simulink model "Sim4_LCL_L_comp_pwm"  (R2019b)
settings: Solver=ode1  StartTime=0.0  StopTime=3  FixedStep=Time_Step  MaxStep=1e-4  RelTol=1e-3
undefined symbols (not defined in the file): GRD00_Lg, GRD00_Rg, Time_Step
libraries: powerlib x13, GFo_Lib x2, Source_Lib x1, powerlib_meascontrol x1
settings Model: Creator=Frederic_Colas  LastModifiedBy=fcolas
settings DataIOCC: ReturnWorkspaceOutputs=off
settings OptimizationCC: LifeSpan=inf
settings DebuggingCC: UnconnectedInputMsg=none  UnconnectedOutputMsg=none  UnconnectedLineMsg=none  SFExecutionAtInitializationDiag=none  ArithmeticOperatorsInVariantConditions=warning
settings HardwareCC: ProdBitPerSizeT=32  ProdBitPerPtrDiffT=32  ProdWordSize=32  ProdHWDeviceType=Specified
settings SFSimCC: SimUseLocalCustomCode=off  CustomCodeUndefinedFunction=UseInterfaceOnly
settings RTWCC: RTWUseLocalCustomCode=off
settings CodeAppCC: StateflowObjectComments=on
settings SimscapeCC: SimscapeNormalizeSystem=off

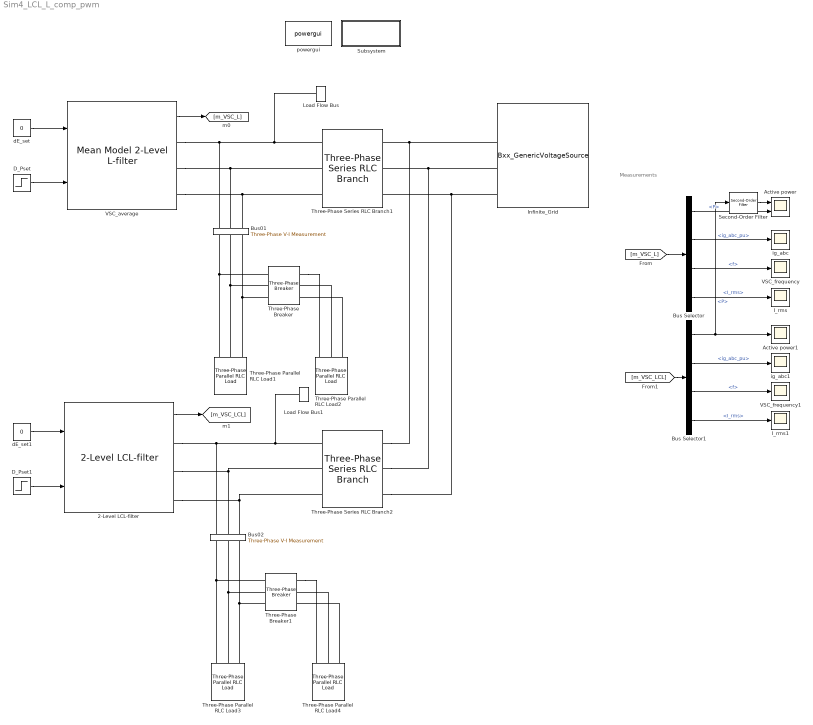
== system Sim4_LCL_L_comp_pwm ==
  note: Measurements
  2-Level LCL-filter : GFo_Lib/2-Level LCL-filter  fn=50  Sn=1000e6  Pn=1000e6  Udcn=640e3  Time_Step=Time_Step  bridge_type=Detailed (switches included)  fpwm=4.33e3  Un1=320e3  Un2=400e3  Rt_pu=0.005  Lt_pu=0.15  Rm_pu=500  Lm_pu=500  Lf_pu=0.15  Rf_pu=0.005  Cf_pu=0.066  H_DC=40  Tr_PLL=10  Val_Freq_Support=on  Val_gamma=on  R_percent=4  Rv=0.09  W_TVR=60  I_thresh_pu=1.2  DX_DR=5  Val_Mod_H=off  RLCL_D=0.7  f_damping=100  I_max_pu=1.2  Tr_I_max=200  Advanced=on  gainpopup=With Inertia  f_Inertia_Less=3  zeta_Inertia_Less=1  Param_Inertia=PI  H_GFo=5  zeta_GFo=1  LFpopup=PQ  P0=0.3  Q0=0  V0=1.0009  Theta0=0.57142
      settings: SourceProductName=VSC4SPS
  Active power : Scope  NumInputPorts=2
  Active power1 : Scope
  Bus Selector : BusSelector  OutputSignals=P,I.ig_abc_pu,f,VI.I_rms
  Bus Selector1 : BusSelector  OutputSignals=P,I.ig_abc_pu,f,VI.I_rms
  "Bus01 " : powerlib/Measurements/Three-Phase V-I Measurement  VoltageMeasurement=no  SetLabelV=off  LabelV=Vabc  Vpu=off  VpuLL=off  CurrentMeasurement=no  SetLabelI=off  LabelI=Iabc  Ipu=off  Pbase=100e6  Vbase=500e3  OutputType=Complex  PhasorSimulation=off  PSBequivalent=0
  Bus02 : powerlib/Measurements/Three-Phase V-I Measurement  VoltageMeasurement=no  SetLabelV=off  LabelV=Vabc  Vpu=off  VpuLL=off  CurrentMeasurement=no  SetLabelI=off  LabelI=Iabc  Ipu=off  Pbase=100e6  Vbase=500e3  OutputType=Complex  PhasorSimulation=off  PSBequivalent=0
  D_Pset : Step  Time=0.25  After=0.6  SampleTime=0
  D_Pset1 : Step  Time=0.25  After=0.6  SampleTime=0
  I_rms : Scope
  I_rms1 : Scope
  Infinite_Grid : Source_Lib/Bxx_GenericVoltageSource  SourceNature_str=INFINITE  fn=50  Sn=1000e6  Un=Ug  Time_Step=0  LFpopup=Swing  P0=-398902388.0153  Q0=3978449.8636  V0_pu=1  U0=20000  Theta0_deg=0  H_s=5  DroopOnOff=on  R_percent=4  TN=1  TD=2
      settings: SourceProductName=VSC4SPS
  Load Flow Bus : powerlib/Measurements/Load Flow Bus  LConnTagsString=a  Phases=single  Connectors=on one side  ID=BUS_1  Vbase=Ug  Vref=1  Vangle=0  VLF=1.001  VLFb=1  VLFc=1  angleLF=0.5714  angleLFb=0  angleLFc=0
  Load Flow Bus1 : powerlib/Measurements/Load Flow Bus  LConnTagsString=a  Phases=single  Connectors=on one side  ID=BUS_2  Vbase=Ug  Vref=1  Vangle=0  VLF=1.001  VLFb=1  VLFc=1  angleLF=0.5714  angleLFb=0  angleLFc=0
  Second-Order Filter : powerlib_meascontrol/Filters/Second-Order Filter  FilterType=Lowpass  Fo=250  Zeta=1  Ts=0  Initialize=on  Vac_Init="[0,  0,  60]"  Vdc_Init=0.3  PlotResponse=off  FreqRange=[0, 500, 1]
      settings: SourceProductBaseCode=PS
  Subsystem : Subsystem
      settings: OpenFcn=LoadFlow_VSC
      mask Display: color('blue'),disp('Update Loadflow')
  Three-Phase Parallel RLC Load1 : powerlib/Elements/Three-Phase Parallel RLC Load  LConnTagsString=A|B|C  Configuration=Y (grounded)  NominalVoltage=Ug  Vabc=[1e3 1e3 1e3]  Vabcp=[1e3 1e3 1e3]  NominalFrequency=fb  UnbalancedPower=off  ActivePower=100e6  InductivePower=0  CapacitivePower=0  Pabc=[10e3 9e3 11e3]  QLabc=[100 90 110]  QCabc=[100 90 110]  Pabcp=[10e3 9e3 11e3]  QLabcp=[100 90 110]  QCabcp=[100 90 110]  Measurements=None  LoadType=constant Z
  Three-Phase Parallel RLC Load2 : powerlib/Elements/Three-Phase Parallel RLC Load  LConnTagsString=A|B|C  Configuration=Y (grounded)  NominalVoltage=Ug  Vabc=[1e3 1e3 1e3]  Vabcp=[1e3 1e3 1e3]  NominalFrequency=fb  UnbalancedPower=off  ActivePower=1000e6  InductivePower=0  CapacitivePower=0  Pabc=[10e3 9e3 11e3]  QLabc=[100 90 110]  QCabc=[100 90 110]  Pabcp=[10e3 9e3 11e3]  QLabcp=[100 90 110]  QCabcp=[100 90 110]  Measurements=None  LoadType=constant Z
  Three-Phase Parallel RLC Load3 : powerlib/Elements/Three-Phase Parallel RLC Load  LConnTagsString=A|B|C  Configuration=Y (grounded)  NominalVoltage=Ug  Vabc=[1e3 1e3 1e3]  Vabcp=[1e3 1e3 1e3]  NominalFrequency=fb  UnbalancedPower=off  ActivePower=100e6  InductivePower=0  CapacitivePower=0  Pabc=[10e3 9e3 11e3]  QLabc=[100 90 110]  QCabc=[100 90 110]  Pabcp=[10e3 9e3 11e3]  QLabcp=[100 90 110]  QCabcp=[100 90 110]  Measurements=None  LoadType=constant Z
  Three-Phase Parallel RLC Load4 : powerlib/Elements/Three-Phase Parallel RLC Load  LConnTagsString=A|B|C  Configuration=Y (grounded)  NominalVoltage=Ug  Vabc=[1e3 1e3 1e3]  Vabcp=[1e3 1e3 1e3]  NominalFrequency=fb  UnbalancedPower=off  ActivePower=1000e6  InductivePower=0  CapacitivePower=0  Pabc=[10e3 9e3 11e3]  QLabc=[100 90 110]  QCabc=[100 90 110]  Pabcp=[10e3 9e3 11e3]  QLabcp=[100 90 110]  QCabcp=[100 90 110]  Measurements=None  LoadType=constant Z
  Three-Phase Series RLC Branch1 : powerlib/Elements/Three-Phase Series RLC Branch  LConnTagsString=A|B|C  RConnTagsString=A|B|C  BranchType=RL  Resistance=GRD00_Rg  Inductance=GRD00_Lg  Capacitance=1e-6  Measurements=None
  Three-Phase Series RLC Branch2 : powerlib/Elements/Three-Phase Series RLC Branch  LConnTagsString=A|B|C  RConnTagsString=A|B|C  BranchType=RL  Resistance=GRD00_Rg  Inductance=GRD00_Lg  Capacitance=1e-6  Measurements=None
  Three-Phase Breaker : powerlib/Elements/Three-Phase Breaker  InitialState=open  SwitchA=on  SwitchB=on  SwitchC=on  SwitchTimes=1  External=off  BreakerResistance=0.01  SnubberResistance=1e6  SnubberCapacitance=inf  Measurements=None
  Three-Phase Breaker1 : powerlib/Elements/Three-Phase Breaker  InitialState=open  SwitchA=on  SwitchB=on  SwitchC=on  SwitchTimes=1  External=off  BreakerResistance=0.01  SnubberResistance=1e6  SnubberCapacitance=inf  Measurements=None
  VSC_average : GFo_Lib/Mean Model 2-Level L-filter  fn=50  Sn=1000e6  Pn=1000e6  Udcn=640e3  Time_Step=Time_Step  Un1=320e3  Un2=Ug  Rt_pu=0.005  Lt_pu=0.15  Lm_pu=500  Rm_pu=500  Tr_PLL=10  Val_Freq_Support=on  R_percent=4  Rv=0.09  W_TVR=60  I_max_VI_pu=1.2  DX_DR=5  Val_Mod_H=off  I_max_pu=1.2  Tr_I_max=200  Advanced=on  gainpopup=With Inertia  f_Inertia_Less=5  zeta_Inertia_Less=1  Param_Inertia=PI  H_GFo=5  zeta_GFo=1  LFpopup=PQ  P0=0.3  Q0=2.3716e-08  V0=1.0009  Theta0=0.57142
      settings: SourceProductName=VSC4SPS
  VSC_frequency : Scope
  VSC_frequency1 : Scope
  dE_set : Constant  Value=0
  dE_set1 : Constant  Value=0
  ig_abc : Scope
  ig_abc1 : Scope
  powergui : powerlib/powergui  Priority=1  SimulationMode=Discrete  SampleTime=Time_Step  frequency=60  Iterations=50  frequencyindice=50  Pbase=1000000000  ErrMax=1e-6  UnitsV=kV  UnitsW=MW  buscounter=0  FunctionMessages=off  echomessages=off  EnableUseOfTLC=off  CurrentSourceSwitches=off  DisableSnubberDevices=off  DisableRonSwitches=off  DisableVfSwitches=off  DisplayEquations=off  AutomaticDiscreteSolvers=off  SolverType=Tustin/Backward Euler (TBE)  Interpol=off  ExternalGateDelay=off  methode=off  Ts=100  x0status=blocks  SPID=on  SwTol=0  HookPort=off  NonlinearTolerance=1e-4  nMaxIteration=100  ContinueOnMaxIteration=off  RestoreLinks=warning  ResistiveCurrentMeasurement=off  Frange=[0:2:500]  Ylog=off  Xlog=on  ShowGrid=off  save=off  variable=ZData  structure=0  ZoomFFT=off  StartTime=0.0  cycles=1  DisplayStyle=1  fundamental=60  FreqAxis=off  MaxFrequency=1000  frequencyindicesteady=1  RmsSteady=1  display=off
  wires:
  dE_set/1 -> VSC_average/1
  D_Pset/1 -> VSC_average/2
  [m_VSC_L] -> Bus Selector/1
  Bus Selector/1 -> Active power/2  "<P>"
  VSC_average/1 -> [m_VSC_L]
  Bus Selector/2 -> ig_abc/1  "<ig_abc_pu>"
  Bus Selector/3 -> VSC_frequency/1  "<f>"
  Bus Selector/4 -> I_rms/1  "<I_rms>"
  D_Pset1/1 -> 2-Level LCL-filter/2
  dE_set1/1 -> 2-Level LCL-filter/1
  2-Level LCL-filter/1 -> [m_VSC_LCL]
  Bus Selector1/1 -> Active power1/1, Second-Order Filter/1  "<P>"
  Bus Selector1/2 -> ig_abc1/1  "<ig_abc_pu>"
  [m_VSC_LCL] -> Bus Selector1/1
  Bus Selector1/4 -> I_rms1/1  "<I_rms>"
  Bus Selector1/3 -> VSC_frequency1/1  "<f>"
  Second-Order Filter/1 -> Active power/1
  connections:
  VSC_average/RConn1 -- "Bus01 "/LConn3 -- Load Flow Bus/LConn1 -- Three-Phase Series RLC Branch1/LConn1
  VSC_average/RConn3 -- "Bus01 "/LConn1 -- Three-Phase Series RLC Branch1/LConn3
  VSC_average/RConn2 -- "Bus01 "/LConn2 -- Three-Phase Series RLC Branch1/LConn2
  Infinite_Grid/RConn1 -- Three-Phase Series RLC Branch2/RConn1 -- Three-Phase Series RLC Branch1/RConn1
  Infinite_Grid/RConn2 -- Three-Phase Series RLC Branch2/RConn2 -- Three-Phase Series RLC Branch1/RConn2
  Infinite_Grid/RConn3 -- Three-Phase Series RLC Branch2/RConn3 -- Three-Phase Series RLC Branch1/RConn3
  Three-Phase Parallel RLC Load1/LConn2 -- Three-Phase Breaker/LConn2 -- "Bus01 "/RConn2
  Three-Phase Parallel RLC Load1/LConn3 -- Three-Phase Breaker/LConn3 -- "Bus01 "/RConn1
  Three-Phase Parallel RLC Load1/LConn1 -- Three-Phase Breaker/LConn1 -- "Bus01 "/RConn3
  Three-Phase Parallel RLC Load2/LConn3 -- Three-Phase Breaker/RConn3
  Three-Phase Parallel RLC Load2/LConn2 -- Three-Phase Breaker/RConn2
  Three-Phase Breaker/RConn1 -- Three-Phase Parallel RLC Load2/LConn1
  Bus02/LConn3 -- 2-Level LCL-filter/RConn1 -- Load Flow Bus1/LConn1 -- Three-Phase Series RLC Branch2/LConn1
  Bus02/LConn2 -- Three-Phase Series RLC Branch2/LConn2 -- 2-Level LCL-filter/RConn2
  Bus02/LConn1 -- Three-Phase Series RLC Branch2/LConn3 -- 2-Level LCL-filter/RConn3
  Three-Phase Breaker1/LConn2 -- Three-Phase Parallel RLC Load3/LConn2 -- Bus02/RConn2
  Three-Phase Breaker1/LConn3 -- Three-Phase Parallel RLC Load3/LConn3 -- Bus02/RConn1
  Three-Phase Breaker1/LConn1 -- Three-Phase Parallel RLC Load3/LConn1 -- Bus02/RConn3
  Three-Phase Parallel RLC Load4/LConn2 -- Three-Phase Breaker1/RConn2
  Three-Phase Parallel RLC Load4/LConn3 -- Three-Phase Breaker1/RConn3
  Three-Phase Breaker1/RConn1 -- Three-Phase Parallel RLC Load4/LConn1

== system Sim4_LCL_L_comp_pwm/Subsystem ==
